simulink model "gm_Both_Test_fil"  (R2016b)
settings: Solver=VariableStepAuto  StartTime=0.0  StopTime=3  RelTol=1e-3
PreLoadFcn:
  | addpath('C:\Users\paul.rogers\OldStuff\GradSchool\MATLAB\Both_Test\hdl_prj\hdlsrc\Both_Test');
undefined symbols (not defined in the file): sigbuilder_block
libraries: powerlib x12, simulink x7, nesl_utility x2, fl_lib x2, fillib x1
settings Model: Creator=paul.rogers  LastModifiedBy=paul.rogers
settings OptimizationCC: BlockReduction=off  ConditionallyExecuteInputs=off  DefaultParameterBehavior=Inlined
settings DebuggingCC: AlgebraicLoopMsg=error  InheritedTsInSrcMsg=none  SingleTaskRateTransMsg=error
settings HardwareCC: ProdBitPerPointer=32  ProdBitPerSizeT=32  ProdBitPerPtrDiffT=32  ProdLargestAtomicFloat=None  ProdIntDivRoundTo=Undefined  ProdEndianess=Unspecified  ProdWordSize=32  ProdHWDeviceType=ASIC/FPGA->ASIC/FPGA  ProdEqTarget=off

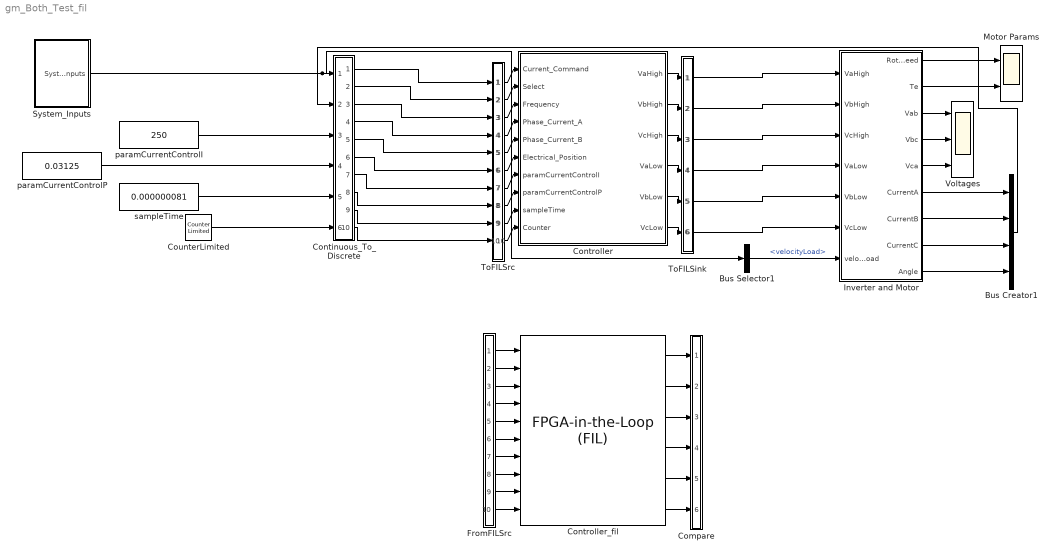
== system gm_Both_Test_fil ==
  Bus Creator1 : BusCreator  Inputs=4
  Bus Selector1 : BusSelector  OutputSignals=velocityLoad
  Compare : Subsystem
      mask Display: disp('')
  Continuous_To_Discrete : Subsystem
      mask Display: fprintf('C/D')
  Controller : Subsystem
  Controller_fil : fillib/FPGA-in-the-Loop (FIL)  ForceInterfaceUpdate=0.91338
  CounterLimited : simulink/Sources/Counter Limited  uplimit=50  tsamp=1e-7
  FromFILSrc : Subsystem
      mask Display: disp('')
  Inverter and Motor : Subsystem
  Motor Params : Scope  NumInputPorts=2
  System_Inputs : Subsystem  Description=""
      mask Display: disp('System\nInputs')
  ToFILSink : Subsystem
      mask Display: disp('')
  ToFILSrc : Subsystem
      mask Display: disp('')
  "Voltages " : Scope  NumInputPorts=3
  paramCurrentControlI : Constant  Value=250  OutDataTypeStr=fixdt(1,16,3)
  paramCurrentControlP : Constant  Value=0.03125  OutDataTypeStr=fixdt(1,16,8)
  sampleTime : Constant  Value=0.000000081  OutDataTypeStr=fixdt(1,16,30)
  wires:
  Inverter and Motor/9(Angle) -> Bus Creator1/4
  Inverter and Motor/8(CurrentC) -> Bus Creator1/3
  Inverter and Motor/6(CurrentA) -> Bus Creator1/1
  Inverter and Motor/7(CurrentB) -> Bus Creator1/2
  paramCurrentControlP/1 -> Continuous_To_Discrete/4(paramCurrentControlP)
  paramCurrentControlI/1 -> Continuous_To_Discrete/3(paramCurrentControlI)
  System_Inputs/1(System_Inputs) -> Bus Selector1/1, Continuous_To_Discrete/1(System_Inputs)
  Bus Creator1/1 -> Continuous_To_Discrete/2(Motor_Measurements)
  sampleTime/1 -> Continuous_To_Discrete/5(sampleTime)
  Bus Selector1/1 -> Inverter and Motor/7(velocityLoad)  "<velocityLoad>"
  Inverter and Motor/2(Te) -> Motor Params/2
  Inverter and Motor/1(Rotor Speed) -> Motor Params/1
  Inverter and Motor/3(Vab) -> "Voltages "/1
  Inverter and Motor/4(Vbc) -> "Voltages "/2
  Inverter and Motor/5(Vca) -> "Voltages "/3
  CounterLimited/1 -> Continuous_To_Discrete/6(Counter)
  ToFILSrc/1(out1) -> Controller/1(Current_Command)
  ToFILSrc/2(out2) -> Controller/2(Select)
  ToFILSrc/3(out3) -> Controller/3(Frequency)
  ToFILSrc/4(out4) -> Controller/4(Phase_Current_A)
  ToFILSrc/5(out5) -> Controller/5(Phase_Current_B)
  ToFILSrc/6(out6) -> Controller/6(Electrical_Position)
  ToFILSrc/7(out7) -> Controller/7(paramCurrentControlI)
  ToFILSrc/8(out8) -> Controller/8(paramCurrentControlP)
  ToFILSrc/9(out9) -> Controller/9(sampleTime)
  ToFILSrc/10(out10) -> Controller/10(Counter)
  Controller/1(VaHigh) -> ToFILSink/1(in1)
  Controller/2(VbHigh) -> ToFILSink/2(in2)
  Controller/3(VcHigh) -> ToFILSink/3(in3)
  Controller/4(VaLow) -> ToFILSink/4(in4)
  Controller/5(VbLow) -> ToFILSink/5(in5)
  Controller/6(VcLow) -> ToFILSink/6(in6)
  Continuous_To_Discrete/1(Current_Command) -> ToFILSrc/1(in1)
  Continuous_To_Discrete/2(Switch) -> ToFILSrc/2(in2)
  Continuous_To_Discrete/3(Frequency) -> ToFILSrc/3(in3)
  Continuous_To_Discrete/4(Phase_Current_A) -> ToFILSrc/4(in4)
  Continuous_To_Discrete/5(Phase_Current_B) -> ToFILSrc/5(in5)
  Continuous_To_Discrete/6(Electrical_Position) -> ToFILSrc/6(in6)
  Continuous_To_Discrete/7(paramCurrentControlI_timed) -> ToFILSrc/7(in7)
  Continuous_To_Discrete/8(paramCurrentControlP_timed) -> ToFILSrc/8(in8)
  Continuous_To_Discrete/9(sampleTime_timed) -> ToFILSrc/9(in9)
  Continuous_To_Discrete/10(Counter_timed) -> ToFILSrc/10(in10)
  ToFILSink/1(out1) -> Inverter and Motor/1(VaHigh)
  ToFILSink/2(out2) -> Inverter and Motor/2(VbHigh)
  ToFILSink/3(out3) -> Inverter and Motor/3(VcHigh)
  ToFILSink/4(out4) -> Inverter and Motor/4(VaLow)
  ToFILSink/5(out5) -> Inverter and Motor/5(VbLow)
  ToFILSink/6(out6) -> Inverter and Motor/6(VcLow)
  FromFILSrc/1(out1) -> Controller_fil/1
  FromFILSrc/2(out2) -> Controller_fil/2
  FromFILSrc/3(out3) -> Controller_fil/3
  FromFILSrc/4(out4) -> Controller_fil/4
  FromFILSrc/5(out5) -> Controller_fil/5
  FromFILSrc/6(out6) -> Controller_fil/6
  FromFILSrc/7(out7) -> Controller_fil/7
  FromFILSrc/8(out8) -> Controller_fil/8
  FromFILSrc/9(out9) -> Controller_fil/9
  FromFILSrc/10(out10) -> Controller_fil/10
  Controller_fil/1 -> Compare/1(in1)
  Controller_fil/2 -> Compare/2(in2)
  Controller_fil/3 -> Compare/3(in3)
  Controller_fil/4 -> Compare/4(in4)
  Controller_fil/5 -> Compare/5(in5)
  Controller_fil/6 -> Compare/6(in6)

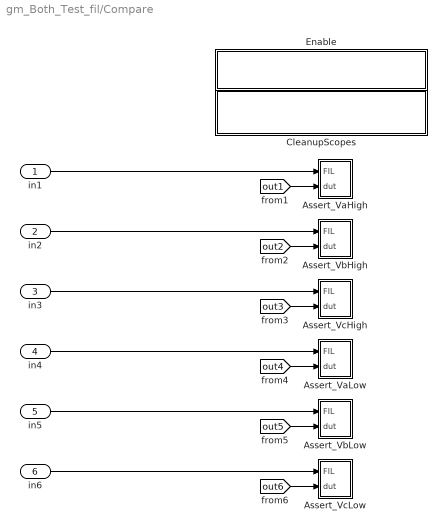
== system gm_Both_Test_fil/Compare ==
  in1 : Inport
  in2 : Inport  Port=2
  in3 : Inport  Port=3
  in4 : Inport  Port=4
  in5 : Inport  Port=5
  in6 : Inport  Port=6
  Assert_VaHigh : Subsystem
  Assert_VaLow : Subsystem
  Assert_VbHigh : Subsystem
  Assert_VbLow : Subsystem
  Assert_VcHigh : Subsystem
  Assert_VcLow : Subsystem
  CleanupScopes : Subsystem
      settings: OpenFcn=|
      | blkName = gcb; %self block
      | idx = regexp(blkName, '/CleanupScopes$', 'once');
      | blkParent = blkName(1:idx-1);
      | blks=find_system(blkParent, 'LookUnderMasks', 'all','blocktype', 'TimeScope');
      | for itr = 1:length(blks)
      | 	 hScopeCfg = get_param(blks{itr},'ScopeConfiguration');
      | 	 hScopeCfg.Visible = ~ hScopeCfg.Visible;
      | end
      | drawnow;
      mask Display: fprintf(message('hdlcoder:cosim:vnl_dblclick').getString());
  Enable : Subsystem
      settings: OpenFcn=|
      | blkName = gcb;
      | idx = regexp(blkName, '/Enable$', 'once');
      | blkParent = blkName(1:idx-1);
      | blks=find_system(blkParent, 'LookUnderMasks', 'all','blocktype', 'Assertion');
      | e = get_param(blks{1}, 'Enabled');
      | if strcmp(e, 'on'), f= 'off';, else, f = 'on';, end
      | for ii=1:length(blks), set_param(blks{ii}, 'Enabled', f);, end
      | set_param(gcb, 'MaskDisplay',['fprintf(message(''hdlcoder:cosim:vnl_dblclick_assertions'',','''',upper(e),'''',').getString())']);
      mask Display: fprintf(message('hdlcoder:cosim:vnl_dblclick_assertions','OFF').getString());
  wires:
  in1/1 -> Assert_VaHigh/1(FIL)
  [out1] -> Assert_VaHigh/2(dut)
  in2/1 -> Assert_VbHigh/1(FIL)
  [out2] -> Assert_VbHigh/2(dut)
  in3/1 -> Assert_VcHigh/1(FIL)
  [out3] -> Assert_VcHigh/2(dut)
  in4/1 -> Assert_VaLow/1(FIL)
  [out4] -> Assert_VaLow/2(dut)
  in5/1 -> Assert_VbLow/1(FIL)
  [out5] -> Assert_VbLow/2(dut)
  in6/1 -> Assert_VcLow/1(FIL)
  [out6] -> Assert_VcLow/2(dut)

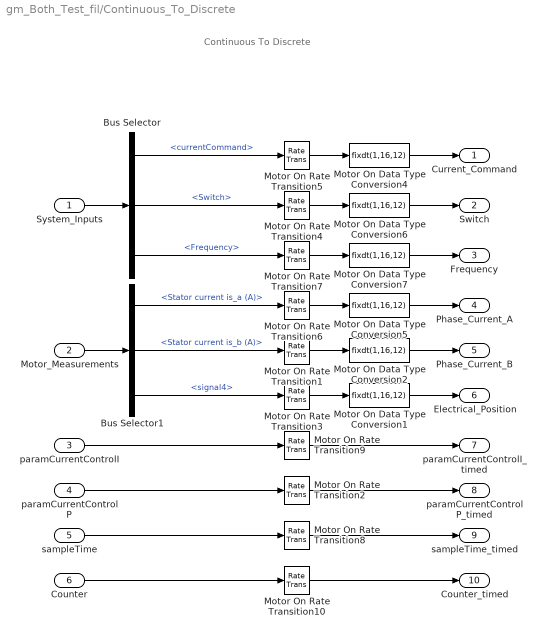
== system gm_Both_Test_fil/Continuous_To_Discrete ==
  note: Continuous To Discrete
  System_Inputs : Inport
  Motor_Measurements : Inport  Port=2
  paramCurrentControlI : Inport  Port=3
  paramCurrentControlP : Inport  Port=4
  sampleTime : Inport  Port=5
  Counter : Inport  Port=6  OutDataTypeStr=uint8
  Bus Selector : BusSelector  OutputSignals=currentCommand,Switch,Frequency
  Bus Selector1 : BusSelector  OutputSignals=Stator current is_a (A),Stator current is_b (A),signal4
  Motor On Data Type Conversion{1..2,4..7} (6 alike) : DataTypeConversion  OutDataTypeStr=fixdt(1,16,12)
  Motor On Rate Transition{1..10} (10 alike) : RateTransition  Integrity=off  Deterministic=off  OutPortSampleTime=0.000000081
  Current_Command : Outport
  Switch : Outport  Port=2
  Frequency : Outport  Port=3
  Phase_Current_A : Outport  Port=4
  Phase_Current_B : Outport  Port=5
  Electrical_Position : Outport  Port=6
  paramCurrentControlI_timed : Outport  Port=7
  paramCurrentControlP_timed : Outport  Port=8
  sampleTime_timed : Outport  Port=9
  Counter_timed : Outport  Port=10
  wires:
  Bus Selector1/3 -> Motor On Rate Transition3/1  "<signal4>"
  Bus Selector1/2 -> Motor On Rate Transition1/1  "<Stator current is_b (A)>"
  Bus Selector1/1 -> Motor On Rate Transition6/1  "<Stator current is_a (A)>"
  Motor On Data Type Conversion4/1 -> Current_Command/1
  Motor On Rate Transition6/1 -> Motor On Data Type Conversion5/1
  Motor On Rate Transition5/1 -> Motor On Data Type Conversion4/1
  Bus Selector/1 -> Motor On Rate Transition5/1  "<currentCommand>"
  Motor On Rate Transition3/1 -> Motor On Data Type Conversion1/1
  System_Inputs/1 -> Bus Selector/1
  Motor_Measurements/1 -> Bus Selector1/1
  Motor On Rate Transition1/1 -> Motor On Data Type Conversion2/1
  Motor On Rate Transition4/1 -> Motor On Data Type Conversion6/1
  Bus Selector/2 -> Motor On Rate Transition4/1  "<Switch>"
  Motor On Rate Transition7/1 -> Motor On Data Type Conversion7/1
  Bus Selector/3 -> Motor On Rate Transition7/1  "<Frequency>"
  Motor On Data Type Conversion6/1 -> Switch/1
  Motor On Data Type Conversion7/1 -> Frequency/1
  Motor On Data Type Conversion1/1 -> Electrical_Position/1
  Motor On Data Type Conversion2/1 -> Phase_Current_B/1
  Motor On Data Type Conversion5/1 -> Phase_Current_A/1
  paramCurrentControlI/1 -> Motor On Rate Transition9/1
  paramCurrentControlP/1 -> Motor On Rate Transition2/1
  sampleTime/1 -> Motor On Rate Transition8/1
  Counter/1 -> Motor On Rate Transition10/1
  Motor On Rate Transition10/1 -> Counter_timed/1
  Motor On Rate Transition8/1 -> sampleTime_timed/1
  Motor On Rate Transition2/1 -> paramCurrentControlP_timed/1
  Motor On Rate Transition9/1 -> paramCurrentControlI_timed/1

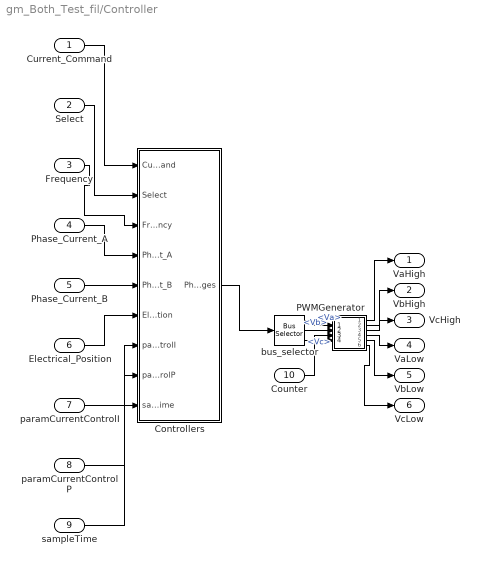
== system gm_Both_Test_fil/Controller ==
  Current_Command : Inport  OutDataTypeStr=fixdt(1, 16, 12)  SampleTime=8.1e-08
  Select : Inport  Port=2  OutDataTypeStr=fixdt(1, 16, 12)  SampleTime=8.1e-08
  Frequency : Inport  Port=3  OutDataTypeStr=fixdt(1, 16, 12)  SampleTime=8.1e-08
  Phase_Current_A : Inport  Port=4  OutDataTypeStr=fixdt(1, 16, 12)  SampleTime=8.1e-08
  Phase_Current_B : Inport  Port=5  OutDataTypeStr=fixdt(1, 16, 12)  SampleTime=8.1e-08
  Electrical_Position : Inport  Port=6  OutDataTypeStr=fixdt(1, 16, 12)  SampleTime=8.1e-08
  paramCurrentControlI : Inport  Port=7  OutDataTypeStr=fixdt(1, 16, 3)  SampleTime=8.1e-08
  paramCurrentControlP : Inport  Port=8  OutDataTypeStr=fixdt(1, 16, 8)  SampleTime=8.1e-08
  sampleTime : Inport  Port=9  OutDataTypeStr=fixdt(1, 16, 30)  SampleTime=8.1e-08
  Counter : Inport  Port=10  OutDataTypeStr=uint8  SampleTime=8.1e-08
  Controllers : Subsystem
  PWMGenerator : ModelReference  ModelNameDialog=gm_PWMGenerator.slx  SimulationMode=Normal  ModelReferenceVersion=1.12
  bus_selector : BusSelector  OutputSignals=Va,Vb,Vc
  VaHigh : Outport
  VbHigh : Outport  Port=2
  VcHigh : Outport  Port=3
  VaLow : Outport  Port=4
  VbLow : Outport  Port=5
  VcLow : Outport  Port=6
  wires:
  PWMGenerator/6 -> VcLow/1
  PWMGenerator/5 -> VbLow/1
  PWMGenerator/4 -> VaLow/1
  PWMGenerator/3 -> VcHigh/1
  PWMGenerator/2 -> VbHigh/1
  PWMGenerator/1 -> VaHigh/1
  Controllers/1(Phase_Voltages) -> bus_selector/1
  bus_selector/3 -> PWMGenerator/3  "<Vc>"
  bus_selector/2 -> PWMGenerator/2  "<Vb>"
  bus_selector/1 -> PWMGenerator/1  "<Va>"
  Counter/1 -> PWMGenerator/4
  sampleTime/1 -> Controllers/9(sampleTime)
  paramCurrentControlP/1 -> Controllers/8(paramCurrentControlP)
  paramCurrentControlI/1 -> Controllers/7(paramCurrentControlI)
  Electrical_Position/1 -> Controllers/6(Electrical_Position)
  Phase_Current_B/1 -> Controllers/5(Phase_Current_B)
  Phase_Current_A/1 -> Controllers/4(Phase_Current_A)
  Frequency/1 -> Controllers/3(Frequency)
  Select/1 -> Controllers/2(Select)
  Current_Command/1 -> Controllers/1(Current_Command)

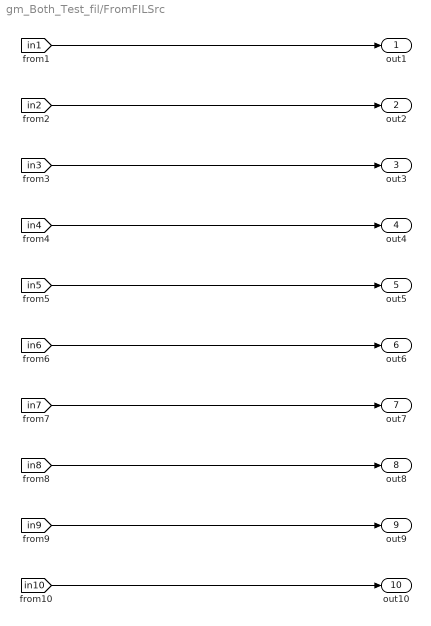
== system gm_Both_Test_fil/FromFILSrc ==
  out1 : Outport
  out2 : Outport  Port=2
  out3 : Outport  Port=3
  out4 : Outport  Port=4
  out5 : Outport  Port=5
  out6 : Outport  Port=6
  out7 : Outport  Port=7
  out8 : Outport  Port=8
  out9 : Outport  Port=9
  out10 : Outport  Port=10
  wires:
  [in1] -> out1/1
  [in2] -> out2/1
  [in3] -> out3/1
  [in4] -> out4/1
  [in5] -> out5/1
  [in6] -> out6/1
  [in7] -> out7/1
  [in8] -> out8/1
  [in9] -> out9/1
  [in10] -> out10/1

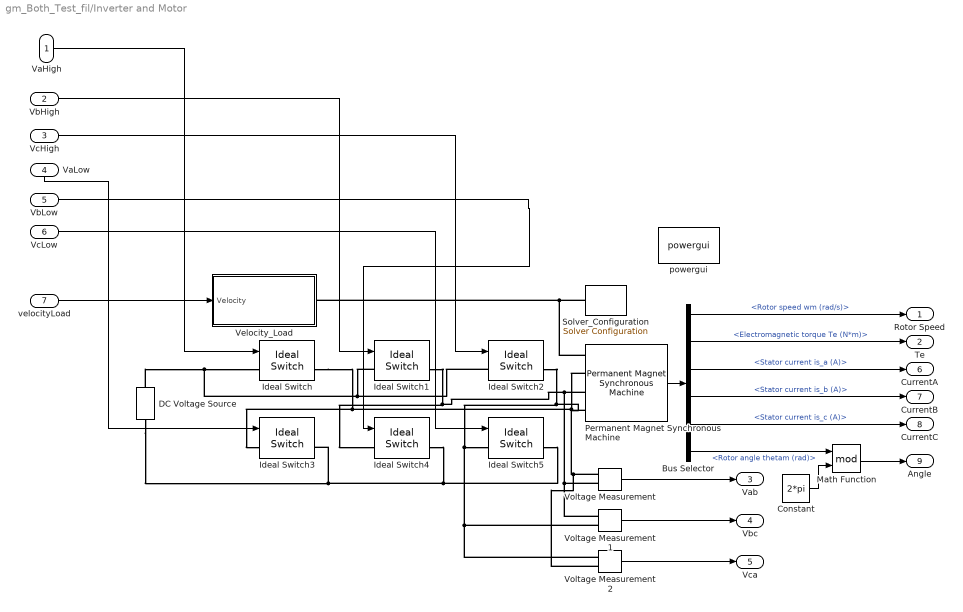
== system gm_Both_Test_fil/Inverter and Motor ==
  VaHigh : Inport
  VbHigh : Inport  Port=2
  VcHigh : Inport  Port=3
  VaLow : Inport  Port=4
  VbLow : Inport  Port=5
  VcLow : Inport  Port=6
  velocityLoad : Inport  Port=7
  Bus Selector : BusSelector  OutputSignals=Rotor speed wm (rad/s),Electromagnetic torque Te (N*m),Stator current is_a (A),Stator current is_b (A),Stator current is_c (A),Rotor angle thetam (rad)
  Constant : Constant  Value=2*pi
  DC Voltage Source : powerlib/Electrical Sources/DC Voltage Source  Amplitude=42  Measurements=None
  Ideal Switch{,1..5} (6 alike) : powerlib/Power Electronics/Ideal Switch  Ron=0.001  Lon=0  IC=0  Rs=1e5  Cs=inf  Measurements=on
  Math Function : Math  Operator=mod  SaturateOnIntegerOverflow=on
  Permanent Magnet Synchronous Machine : powerlib/Machines/Permanent Magnet Synchronous Machine  NbPhases=3  FluxDistribution=Sinusoidal  RotorType=Round  MechanicalLoad=Mechanical rotational port  PresetModel=No  ShowDetailedParameters=on  MeasurementBus=off  Resistance=0.095  Inductance=8.5e-3  dqInductances=[0.000528 0.000655]  La=0.00049  MachineConstant=Flux linkage established by magnets (V.s)  Flux=0.0100933  VoltageCst=9.1536  TorqueCst=0.0757  Flat=120  Mechanical=[0.000621417 0.000303448 5]  PolePairs=4  InitialConditions=[0,0, 0,0]  InitialConditions5ph=[0 0 0 0 0 0]  TsPowergui=0  TsBlock=-1  RefAngle=90 degrees behind phase A axis (modified Park)
  Solver_Configuration : nesl_utility/Solver Configuration  PhysicalDomain=network_engine_domain  SubClassName=solver  LeftPortType=input  RightPortType=generic  Accelerate=off  Tones=[]  Harmonics=[]  SimulateNoise=off  Profile=off  UseLocalSampling=off  EnableSwitchedLinearOptims=on  FrequencyDomain=off  UseCCode=off  RelTol=0.001  AbsTol=1e-06  MinStep=1e-09  ToWorkspace=off  RevertToSquareIcSolve=off  NumHomotopyIterations=100  PhasorMode=off  PhasorModeNumHarmonics=1  OverrideAbsTol=off  DoDC=off  ResidualTolerance=1e-9  UseLocalSolver=off  LocalSolverChoice=NE_BACKWARD_EULER_ADVANCER  LocalSolverSampleTime=.001  DoFixedCost=off  MaxNonlinIter=3  MaxModeIter=2  LinearAlgebra=Sparse  DelaysMemoryBudget=1024  AutomaticFiltering=on  FilteringTimeConstant=0.001
  Velocity_Load : Subsystem  VariantControl=loadType == motorLoad.disc
      mask Display:
      | image('hdlcoderVelocityLoadMask.png')
      | text(0.03, 0.5, '\omega', 'HorizontalAlignment', 'Left', 'texmode','on')
      | text(0.98, 0.5, 'R', 'HorizontalAlignment', 'Right')
  Voltage Measurement : powerlib/Measurements/Voltage Measurement  PhasorSimulation=off  OutputType=Complex  PSBequivalent=0
  Voltage Measurement1 : powerlib/Measurements/Voltage Measurement  PhasorSimulation=off  OutputType=Complex  PSBequivalent=0
  Voltage Measurement2 : powerlib/Measurements/Voltage Measurement  PhasorSimulation=off  OutputType=Complex  PSBequivalent=0
  powergui : powerlib/powergui  Priority=1  SimulationMode=Continuous  SolverType=Tustin/Backward Euler (TBE)  SampleTime=50e-6  frequency=60  SPID=on  DisableSnubberDevices=off  DisableRonSwitches=off  DisableVfSwitches=off  SwTol=0  DisplayEquations=off  Interpol=off  ExternalGateDelay=off  methode=off  Ts=10  FunctionMessages=off  echomessages=off  HookPort=off  EnableUseOfTLC=off  x0status=blocks  frequencyindice=0  Pbase=100e6  ErrMax=1e-4  Iterations=50  UnitsV=kV  UnitsW=MW  buscounter=0  RestoreLinks=warning  ResistiveCurrentMeasurement=off  Frange=[0:2:500]  Ylog=off  Xlog=on  ShowGrid=off  save=off  variable=ZData  structure=0  ZoomFFT=off  StartTime=0.0  cycles=1  DisplayStyle=1  fundamental=60  FreqAxis=off  MaxFrequency=1000  frequencyindicesteady=1  RmsSteady=1  display=off
  Rotor Speed : Outport
  Te : Outport  Port=2
  Vab : Outport  Port=3
  Vbc : Outport  Port=4
  Vca : Outport  Port=5
  CurrentA : Outport  Port=6
  CurrentB : Outport  Port=7
  CurrentC : Outport  Port=8
  Angle : Outport  Port=9
  wires:
  VbHigh/1 -> Ideal Switch1/1
  VcHigh/1 -> Ideal Switch2/1
  VcLow/1 -> Ideal Switch5/1
  VbLow/1 -> Ideal Switch4/1
  Permanent Magnet Synchronous Machine/1 -> Bus Selector/1
  Bus Selector/1 -> Rotor Speed/1  "<Rotor speed wm (rad/s)>"
  Bus Selector/2 -> Te/1  "<Electromagnetic torque Te (N*m)>"
  VaHigh/1 -> Ideal Switch/1
  Voltage Measurement2/1 -> Vca/1
  Voltage Measurement/1 -> Vab/1
  Voltage Measurement1/1 -> Vbc/1
  VaLow/1 -> Ideal Switch3/1
  Bus Selector/3 -> CurrentA/1  "<Stator current is_a (A)>"
  Bus Selector/4 -> CurrentB/1  "<Stator current is_b (A)>"
  Bus Selector/5 -> CurrentC/1  "<Stator current is_c (A)>"
  Bus Selector/6 -> Math Function/1  "<Rotor angle thetam (rad)>"
  Math Function/1 -> Angle/1
  Constant/1 -> Math Function/2
  velocityLoad/1 -> Velocity_Load/1(Velocity)
  connections:
  DC Voltage Source/RConn1 -- Ideal Switch2/LConn1 -- Ideal Switch1/LConn1 -- Ideal Switch/LConn1
  Ideal Switch2/RConn1 -- Permanent Magnet Synchronous Machine/LConn4 -- Voltage Measurement1/LConn2 -- Voltage Measurement2/LConn1 -- Ideal Switch5/LConn1
  Ideal Switch1/RConn1 -- Voltage Measurement/LConn2 -- Voltage Measurement1/LConn1 -- Permanent Magnet Synchronous Machine/LConn3 -- Ideal Switch4/LConn1
  Ideal Switch/RConn1 -- Voltage Measurement2/LConn2 -- Voltage Measurement/LConn1 -- Permanent Magnet Synchronous Machine/LConn2 -- Ideal Switch3/LConn1
  DC Voltage Source/LConn1 -- Ideal Switch5/RConn1 -- Ideal Switch4/RConn1 -- Ideal Switch3/RConn1
  Solver_Configuration/RConn1 -- Permanent Magnet Synchronous Machine/LConn1 -- Velocity_Load/RConn1

== system gm_Both_Test_fil/System_Inputs ==
  note: System Inputs
  Bus Creator : BusCreator  Inputs=4
  Signal_Builder_Experiments : Subsystem  Tag=STV Subsys  LoadFcn=sigbuilder_block('load',[6 30 1428 682.5 ]);  StartFcn=sigbuilder_block('start');  StopFcn=sigbuilder_block('stop');  ClipboardFcn=sigbuilder_block('clipboard');  mask(Sigbuilder block){tuvar=[0:10]}
      mask init:
      | if ~strcmp(get_param(bdroot(gcb),'SimulationStatus'),'stopped'),tuvar = sigbuilder_block('maskInit'); end
      settings: CopyFcn=sigbuilder_block('copy');  DeleteFcn=sigbuilder_block('delete');  ModelCloseFcn=sigbuilder_block('modelClose');  PreSaveFcn=sigbuilder_block('preSave');  PauseFcn=sigbuilder_block('pause');  ContinueFcn=sigbuilder_block('continue');  NameChangeFcn=sigbuilder_block('namechange');  OpenFcn=sigbuilder_block('open',[6 30 1428 682.5 ]);  CloseFcn=sigbuilder_block('close');
      mask Display: plot(0, 0, 100, 100,[2, 2, 32, 32, 2], [68, 8, 8, 68, 68],[32, 2], [38, 38], [32, 19, 2],[53, 60, 44], [32, 17, 17, 2],[16, 16, 31, 31]);txt = getActiveGroup(gcbh);text(2, 100, txt,'verticalAlignment', 'top');
  System_Inputs : Outport
  wires:
  Signal_Builder_Experiments/2(velocityLoad (rad/sec)) -> Bus Creator/2  "velocityLoad"
  Signal_Builder_Experiments/1(currentCommand (Ampere)) -> Bus Creator/1  "currentCommand"
  Bus Creator/1 -> System_Inputs/1
  Signal_Builder_Experiments/3(Switch) -> Bus Creator/3  "Switch"
  Signal_Builder_Experiments/4(Frequency) -> Bus Creator/4  "Frequency"

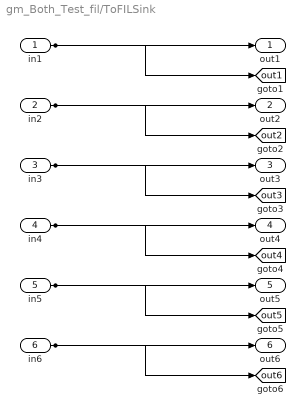
== system gm_Both_Test_fil/ToFILSink ==
  in1 : Inport
  in2 : Inport  Port=2
  in3 : Inport  Port=3
  in4 : Inport  Port=4
  in5 : Inport  Port=5
  in6 : Inport  Port=6
  out1 : Outport
  out2 : Outport  Port=2
  out3 : Outport  Port=3
  out4 : Outport  Port=4
  out5 : Outport  Port=5
  out6 : Outport  Port=6
  tag scope: out1=global, out2=global, out3=global, out4=global, out5=global, out6=global
  wires:
  in1/1 -> out1/1, [out1]
  in2/1 -> out2/1, [out2]
  in3/1 -> out3/1, [out3]
  in4/1 -> out4/1, [out4]
  in5/1 -> out5/1, [out5]
  in6/1 -> out6/1, [out6]

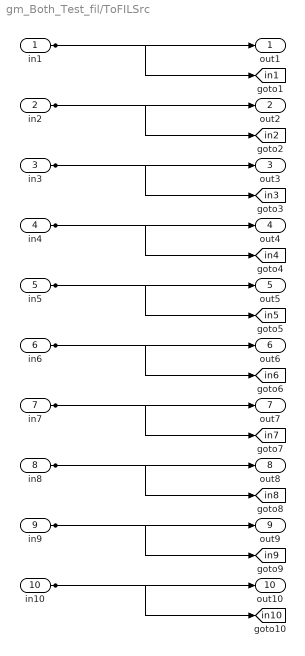
== system gm_Both_Test_fil/ToFILSrc ==
  in1 : Inport
  in2 : Inport  Port=2
  in3 : Inport  Port=3
  in4 : Inport  Port=4
  in5 : Inport  Port=5
  in6 : Inport  Port=6
  in7 : Inport  Port=7
  in8 : Inport  Port=8
  in9 : Inport  Port=9
  in10 : Inport  Port=10
  out1 : Outport
  out2 : Outport  Port=2
  out3 : Outport  Port=3
  out4 : Outport  Port=4
  out5 : Outport  Port=5
  out6 : Outport  Port=6
  out7 : Outport  Port=7
  out8 : Outport  Port=8
  out9 : Outport  Port=9
  out10 : Outport  Port=10
  tag scope: in10=global, in1=global, in2=global, in3=global, in4=global, in5=global, in6=global, in7=global, in8=global, in9=global
  wires:
  in1/1 -> out1/1, [in1]
  in2/1 -> out2/1, [in2]
  in3/1 -> out3/1, [in3]
  in4/1 -> out4/1, [in4]
  in5/1 -> out5/1, [in5]
  in6/1 -> out6/1, [in6]
  in7/1 -> out7/1, [in7]
  in8/1 -> out8/1, [in8]
  in9/1 -> out9/1, [in9]
  in10/1 -> out10/1, [in10]

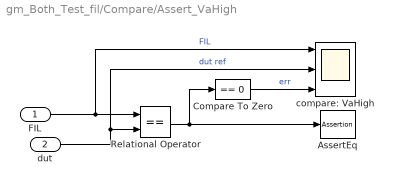
== system gm_Both_Test_fil/Compare/Assert_VaHigh ==
  FIL : Inport
  dut : Inport  Port=2
  AssertEq : Assertion  StopWhenAssertionFail=off
  Compare To Zero : simulink/Logic and Bit Operations/Compare To Zero  relop===  OutDataTypeStr=boolean
  Relational Operator : RelationalOperator  Operator===  OutDataTypeStr=boolean  RndMeth=Nearest
  compare: VaHigh : Scope  NumInputPorts=3
  wires:
  Compare To Zero/1 -> compare: VaHigh/3  "err"
  Relational Operator/1 -> Compare To Zero/1, AssertEq/1
  FIL/1 -> compare: VaHigh/1, Relational Operator/1  "FIL"
  dut/1 -> compare: VaHigh/2, Relational Operator/2  "dut ref"

== system gm_Both_Test_fil/Compare/Assert_VaLow ==
  FIL : Inport
  dut : Inport  Port=2
  AssertEq : Assertion  StopWhenAssertionFail=off
  Compare To Zero : simulink/Logic and Bit Operations/Compare To Zero  relop===  OutDataTypeStr=boolean
  Relational Operator : RelationalOperator  Operator===  OutDataTypeStr=boolean  RndMeth=Nearest
  compare: VaLow : Scope  NumInputPorts=3
  wires:
  Compare To Zero/1 -> compare: VaLow/3  "err"
  Relational Operator/1 -> Compare To Zero/1, AssertEq/1
  FIL/1 -> compare: VaLow/1, Relational Operator/1  "FIL"
  dut/1 -> compare: VaLow/2, Relational Operator/2  "dut ref"

== system gm_Both_Test_fil/Compare/Assert_VbHigh ==
  FIL : Inport
  dut : Inport  Port=2
  AssertEq : Assertion  StopWhenAssertionFail=off
  Compare To Zero : simulink/Logic and Bit Operations/Compare To Zero  relop===  OutDataTypeStr=boolean
  Relational Operator : RelationalOperator  Operator===  OutDataTypeStr=boolean  RndMeth=Nearest
  compare: VbHigh : Scope  NumInputPorts=3
  wires:
  Compare To Zero/1 -> compare: VbHigh/3  "err"
  Relational Operator/1 -> Compare To Zero/1, AssertEq/1
  FIL/1 -> compare: VbHigh/1, Relational Operator/1  "FIL"
  dut/1 -> compare: VbHigh/2, Relational Operator/2  "dut ref"

== system gm_Both_Test_fil/Compare/Assert_VbLow ==
  FIL : Inport
  dut : Inport  Port=2
  AssertEq : Assertion  StopWhenAssertionFail=off
  Compare To Zero : simulink/Logic and Bit Operations/Compare To Zero  relop===  OutDataTypeStr=boolean
  Relational Operator : RelationalOperator  Operator===  OutDataTypeStr=boolean  RndMeth=Nearest
  compare: VbLow : Scope  NumInputPorts=3
  wires:
  Compare To Zero/1 -> compare: VbLow/3  "err"
  Relational Operator/1 -> Compare To Zero/1, AssertEq/1
  FIL/1 -> compare: VbLow/1, Relational Operator/1  "FIL"
  dut/1 -> compare: VbLow/2, Relational Operator/2  "dut ref"

== system gm_Both_Test_fil/Compare/Assert_VcHigh ==
  FIL : Inport
  dut : Inport  Port=2
  AssertEq : Assertion  StopWhenAssertionFail=off
  Compare To Zero : simulink/Logic and Bit Operations/Compare To Zero  relop===  OutDataTypeStr=boolean
  Relational Operator : RelationalOperator  Operator===  OutDataTypeStr=boolean  RndMeth=Nearest
  compare: VcHigh : Scope  NumInputPorts=3
  wires:
  Compare To Zero/1 -> compare: VcHigh/3  "err"
  Relational Operator/1 -> Compare To Zero/1, AssertEq/1
  FIL/1 -> compare: VcHigh/1, Relational Operator/1  "FIL"
  dut/1 -> compare: VcHigh/2, Relational Operator/2  "dut ref"

== system gm_Both_Test_fil/Compare/Assert_VcLow ==
  FIL : Inport
  dut : Inport  Port=2
  AssertEq : Assertion  StopWhenAssertionFail=off
  Compare To Zero : simulink/Logic and Bit Operations/Compare To Zero  relop===  OutDataTypeStr=boolean
  Relational Operator : RelationalOperator  Operator===  OutDataTypeStr=boolean  RndMeth=Nearest
  compare: VcLow : Scope  NumInputPorts=3
  wires:
  Compare To Zero/1 -> compare: VcLow/3  "err"
  Relational Operator/1 -> Compare To Zero/1, AssertEq/1
  FIL/1 -> compare: VcLow/1, Relational Operator/1  "FIL"
  dut/1 -> compare: VcLow/2, Relational Operator/2  "dut ref"

== system gm_Both_Test_fil/Compare/CleanupScopes ==

== system gm_Both_Test_fil/Compare/Enable ==

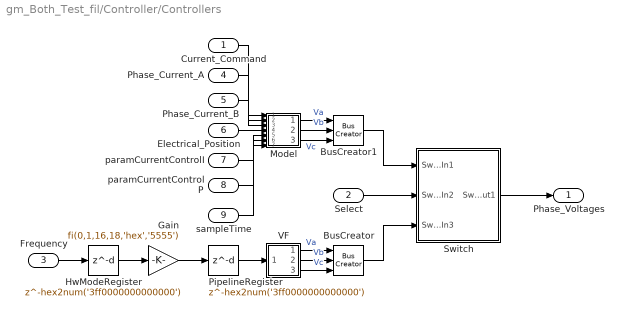
== system gm_Both_Test_fil/Controller/Controllers ==
  Current_Command : Inport  SampleTime=8.1e-08
  Select : Inport  Port=2  SampleTime=8.1e-08
  Frequency : Inport  Port=3  SampleTime=8.1e-08
  Phase_Current_A : Inport  Port=4  SampleTime=8.1e-08
  Phase_Current_B : Inport  Port=5  SampleTime=8.1e-08
  Electrical_Position : Inport  Port=6  SampleTime=8.1e-08
  paramCurrentControlI : Inport  Port=7  SampleTime=8.1e-08
  paramCurrentControlP : Inport  Port=8  SampleTime=8.1e-08
  sampleTime : Inport  Port=9  SampleTime=8.1e-08
  BusCreator : BusCreator  Inputs=3
  BusCreator1 : BusCreator  Inputs=3
  Gain : Gain  Gain=fi(0,1,16,18,'hex','5555')  ParamDataTypeStr=fixdt(1, 16, 18)  OutDataTypeStr=fixdt(1, 16, 12)  SampleTime=8.1e-08
  HwModeRegister : Delay  DelayLength=hex2num('3ff0000000000000')  InitialCondition=0  InputProcessing=Inherited  SampleTime=8.1e-08
  Model : ModelReference  ModelNameDialog=gm_FOC_Modified.slx  SimulationMode=Normal  ModelReferenceVersion=1.65
  PipelineRegister : Delay  DelayLength=hex2num('3ff0000000000000')  InitialCondition=0  InputProcessing=Inherited  SampleTime=8.1e-08
  Switch : Subsystem
  VF : ModelReference  ModelNameDialog=gm_VF.slx  SimulationMode=Normal  ModelReferenceVersion=1.51
  Phase_Voltages : Outport
  wires:
  HwModeRegister/1 -> Gain/1
  Gain/1 -> PipelineRegister/1
  sampleTime/1 -> Model/7
  paramCurrentControlP/1 -> Model/6
  paramCurrentControlI/1 -> Model/5
  Electrical_Position/1 -> Model/4
  Phase_Current_B/1 -> Model/3
  Phase_Current_A/1 -> Model/2
  Frequency/1 -> HwModeRegister/1
  Select/1 -> Switch/2(Switch_In2)
  Current_Command/1 -> Model/1
  VF/3 -> BusCreator/3  "Vc"
  VF/2 -> BusCreator/2  "Vb"
  VF/1 -> BusCreator/1  "Va"
  Switch/1(Switch_Out1) -> Phase_Voltages/1
  Model/3 -> BusCreator1/3  "Vc"
  Model/2 -> BusCreator1/2  "Vb"
  Model/1 -> BusCreator1/1  "Va"
  PipelineRegister/1 -> VF/1
  BusCreator1/1 -> Switch/1(Switch_In1)
  BusCreator/1 -> Switch/3(Switch_In3)

== system gm_Both_Test_fil/Inverter and Motor/Velocity_Load ==
  note: Velocity Load
  Velocity : Inport
  Ideal_Angular_Velocity_Source : fl_lib/Mechanical/Mechanical Sources/Ideal Angular Velocity Source
  Mechanical_Rotational_Reference : fl_lib/Mechanical/Rotational Elements/Mechanical Rotational Reference
  Simulink-PS Converter : nesl_utility/Simulink-PS Converter  PhysicalDomain=network_engine_domain  SubClassName=ps_input  LeftPortType=input  RightPortType=output  PseudoPeriodic=off  Frequencies=[]  NoiseDistribution=none  NoiseParameters=[]  Unit=rad/s  AffineConversion=off  InputFiltering=on  SimscapeFilterOrder=1  InputFilterTimeConstant=.001  UdotUserProvided=1
  R : PMIOPort  Port=1  Side=Right
  wires:
  Velocity/1 -> Simulink-PS Converter/1
  connections:
  Ideal_Angular_Velocity_Source/LConn1 -- R/RConn1
  Simulink-PS Converter/RConn1 -- Ideal_Angular_Velocity_Source/RConn1
  Mechanical_Rotational_Reference/LConn1 -- Ideal_Angular_Velocity_Source/RConn2

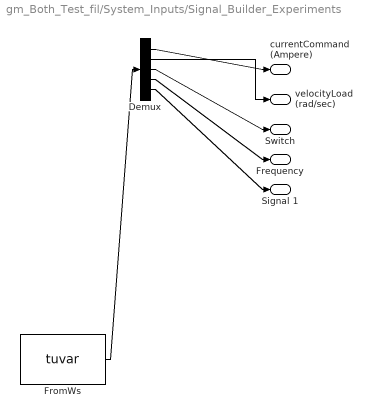
== system gm_Both_Test_fil/System_Inputs/Signal_Builder_Experiments ==
  Demux : Demux  Tag=STV Demux  Outputs=5
  FromWs : FromWorkspace  Tag=STV FromWs  VariableName=tuvar  SampleTime=0
      SigBuilderData=|
      | dataSet(1).timeRange = [0 3]
      | dataSet(1).name = '1 Amp step, locked rotor'
      | dataSet(2).timeRange = [0 3]
      | dataSet(2).name = '+/-1 Amp step, locked rotor'
      | dataSet(3).timeRange = [0 3]
      | dataSet(3).name = '1 Amp, +/-100 rad/sec step'
      | sbobj.Name = 'Signal Builder'
      | sbobj.Groups(1).Name = '1 Amp step, locked rotor'
      | sbobj.Groups(1).Signals(1).Name = 'currentCommand (Ampere)'
      | sbobj.Groups(1).Signals(1).XData = [0 0.05 0.05 0.8 0.8 3]
      | sbobj.Groups(1).Signals(1).YData = [0 0 1 1 0 0]
      | sbobj.Groups(1).Signals(2).Name = 'velocityLoad (rad/sec)'
      | sbobj.Groups(1).Signals(2).XData = [0 3]
      | sbobj.Groups(1).Signals(2).YData = [0 0]
      | sbobj.Groups(1).Signals(3).Name = 'Switch'
      | sbobj.Groups(1).Signals(3).XData = [0 0.5 0.5 3]
      | sbobj.Groups(1).Signals(3).YData = [0 0 1 1]
      | sbobj.Groups(1).Signals(4).Name = 'Frequency'
      | sbobj.Groups(1).Signals(4).XData = [0 3]
      | sbobj.Groups(1).Signals(4).YData = [0 0]
      | sbobj.Groups(1).Signals(5).Name = 'Signal 1'
      | sbobj.Groups(1).Signals(5).XData = [0 1.5 1.5 3]
      | sbobj.Groups(1).Signals(5).YData = [0 0 1 1]
      | sbobj.Groups(1).TimeRange = [0 3]
      | sbobj.Groups(2).Name = '+/-1 Amp step, locked rotor'
      | sbobj.Groups(2).Signals(1).Name = 'currentCommand (Ampere)'
      | sbobj.Groups(2).Signals(1).XData = [0 0.05 0.05 0.5 0.5 0.8 0.8 3]
      | sbobj.Groups(2).Signals(1).YData = [0 0 1 1 -1 -1 0 0]
      | sbobj.Groups(2).Signals(2).Name = 'velocityLoad (rad/sec)'
      | sbobj.Groups(2).Signals(2).XData = [0 1 3]
      | sbobj.Groups(2).Signals(2).YData = [0 0 0]
      | sbobj.Groups(2).Signals(3).Name = 'Switch'
      | sbobj.Groups(2).Signals(3).XData = [0 0.5 0.5 3]
      | sbobj.Groups(2).Signals(3).YData = [0 0 1 1]
      | sbobj.Groups(2).Signals(4).Name = 'Frequency'
      | sbobj.Groups(2).Signals(4).XData = [0 3]
      | sbobj.Groups(2).Signals(4).YData = [0 0]
      | sbobj.Groups(2).Signals(5).Name = 'Signal 1'
      | sbobj.Groups(2).Signals(5).XData = [0 1.5 1.5 3]
      | sbobj.Groups(2).Signals(5).YData = [0 0 1 1]
      | sbobj.Groups(2).TimeRange = [0 3]
      | sbobj.Groups(3).Name = '1 Amp, +/-100 rad/sec step'
      | sbobj.Groups(3).Signals(1).Name = 'currentCommand (Ampere)'
      | sbobj.Groups(3).Signals(1).XData = [0 3]
      | sbobj.Groups(3).Signals(1).YData = [1 1]
      | sbobj.Groups(3).Signals(2).Name = 'velocityLoad (rad/sec)'
      | sbobj.Groups(3).Signals(2).XData = [0 0.5 0.5 1.5 1.5 3]
      | sbobj.Groups(3).Signals(2).YData = [50 50 100 100 50 50]
      | sbobj.Groups(3).Signals(3).Name = 'Switch'
      | sbobj.Groups(3).Signals(3).XData = [0 1 1 3]
      | sbobj.Groups(3).Signals(3).YData = [2 2 0 0]
      | sbobj.Groups(3).Signals(4).Name = 'Frequency'
      | sbobj.Groups(3).Signals(4).XData = [0 1.5 1.5 3]
      | sbobj.Groups(3).Signals(4).YData = [100 100 50 50]
      | sbobj.Groups(3).Signals(5).Name = 'Signal 1'
      | sbobj.Groups(3).Signals(5).XData = [0 1.5 1.5 3]
      | sbobj.Groups(3).Signals(5).YData = [0 0 1 1]
      | sbobj.Groups(3).TimeRange = [0 3]
  currentCommand (Ampere) : Outport  Tag=STV Outport
  velocityLoad (rad/sec) : Outport  Tag=STV Outport  Port=2
  Switch : Outport  Tag=STV Outport  Port=3
  Frequency : Outport  Tag=STV Outport  Port=4
  Signal 1 : Outport  Tag=STV Outport  Port=5
  wires:
  Demux/2 -> velocityLoad (rad/sec)/1
  Demux/1 -> currentCommand (Ampere)/1
  FromWs/1 -> Demux/1
  Demux/3 -> Switch/1
  Demux/4 -> Frequency/1
  Demux/5 -> Signal 1/1

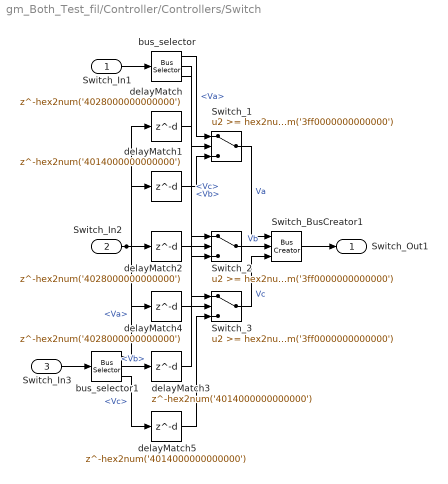
== system gm_Both_Test_fil/Controller/Controllers/Switch ==
  Switch_In1 : Inport  SampleTime=8.1e-08
  Switch_In2 : Inport  Port=2  SampleTime=8.1e-08
  Switch_In3 : Inport  Port=3  SampleTime=8.1e-08
  Switch_1 : Switch  Threshold=hex2num('3ff0000000000000')  OutDataTypeStr=fixdt(1, 84, 66)  SampleTime=8.1e-08
  Switch_2 : Switch  Threshold=hex2num('3ff0000000000000')  OutDataTypeStr=fixdt(1, 84, 66)  SampleTime=8.1e-08
  Switch_3 : Switch  Threshold=hex2num('3ff0000000000000')  OutDataTypeStr=fixdt(1, 84, 66)  SampleTime=8.1e-08
  Switch_BusCreator1 : BusCreator  Inputs=3
  bus_selector : BusSelector  OutputSignals=Va,Vb,Vc
  bus_selector1 : BusSelector  OutputSignals=Va,Vb,Vc
  delayMatch : Delay  DelayLength=hex2num('4028000000000000')  InitialCondition=0  InputProcessing=Inherited  SampleTime=8.1e-08
  delayMatch1 : Delay  DelayLength=hex2num('4014000000000000')  InitialCondition=0  InputProcessing=Inherited  SampleTime=8.1e-08
  delayMatch2 : Delay  DelayLength=hex2num('4028000000000000')  InitialCondition=0  InputProcessing=Inherited  SampleTime=8.1e-08
  delayMatch3 : Delay  DelayLength=hex2num('4014000000000000')  InitialCondition=0  InputProcessing=Inherited  SampleTime=8.1e-08
  delayMatch4 : Delay  DelayLength=hex2num('4028000000000000')  InitialCondition=0  InputProcessing=Inherited  SampleTime=8.1e-08
  delayMatch5 : Delay  DelayLength=hex2num('4014000000000000')  InitialCondition=0  InputProcessing=Inherited  SampleTime=8.1e-08
  Switch_Out1 : Outport
  wires:
  bus_selector1/3 -> delayMatch5/1  "<Vc>"
  bus_selector1/2 -> delayMatch3/1  "<Vb>"
  delayMatch4/1 -> Switch_3/2
  bus_selector1/1 -> delayMatch1/1  "<Va>"
  delayMatch2/1 -> Switch_2/2
  Switch_In3/1 -> bus_selector1/1
  Switch_In2/1 -> delayMatch/1, delayMatch2/1, delayMatch4/1
  Switch_In1/1 -> bus_selector/1
  delayMatch5/1 -> Switch_3/3
  delayMatch3/1 -> Switch_2/3
  delayMatch1/1 -> Switch_1/3
  bus_selector/3 -> Switch_3/1  "<Vc>"
  bus_selector/2 -> Switch_2/1  "<Vb>"
  bus_selector/1 -> Switch_1/1  "<Va>"
  Switch_BusCreator1/1 -> Switch_Out1/1
  Switch_3/1 -> Switch_BusCreator1/3  "Vc"
  Switch_2/1 -> Switch_BusCreator1/2  "Vb"
  Switch_1/1 -> Switch_BusCreator1/1  "Va"
  delayMatch/1 -> Switch_1/2
